simulink model "X-direction-works-UDP"  (R2017a)
settings: Solver=FixedStepDiscrete  StartTime=0.0  StopTime=10.0  FixedStep=0.0002  RelTol=1e-3
libraries: stellaris_lp_lib x7, xpcutilitieslib x2, dspswit3 x1, simulink x1
settings Model: ExtModeTrigDuration=8  Creator=peselnikmg  LastModifiedBy=Rorro
settings DataIOCC: LimitDataPoints=on  SaveFormat=Array  SignalLoggingSaveFormat=ModelDataLogs  ReturnWorkspaceOutputs=on
settings OptimizationCC: UseDivisionForNetSlopeComputation=on  UseFloatMulNetSlope=on  DefaultUnderspecifiedDataType=single  UseSpecifiedMinMax=on  PassReuseOutputArgsAs=Individual arguments  ExpressionDepthLimit=2147483647  ZeroExternalMemoryAtStartup=off  NoFixptDivByZeroProtection=on  EfficientFloat2IntCast=on  LifeSpan=inf  MaxStackSize=64  OptimizeBlockOrder=speed
settings DebuggingCC: ReadBeforeWriteMsg=DisableAll  WriteAfterWriteMsg=DisableAll  WriteAfterReadMsg=DisableAll  MultiTaskDSMMsg=none  IntegerOverflowMsg=error  ParameterTunabilityLossMsg=error  AssertControl=DisableAll  StateNameClashWarn=warning  NonBusSignalsTreatedAsBus=error  SFInvalidInputDataAccessInChartInitDiag=error  SFTransitionOutsideNaturalParentDiag=error  SFUnreachableExecutionPathDiag=error  SFUndirectedBroadcastEventsDiag=error  SFExecutionAtInitializationDiag=none  IntegerSaturationMsg=error
settings HardwareCC: ProdBitPerPointer=32  ProdBitPerSizeT=32  ProdBitPerPtrDiffT=32  ProdLargestAtomicInteger=Long  ProdLargestAtomicFloat=Double  ProdWordSize=32  ProdHWDeviceType=ARM Compatible->ARM Cortex
settings ModelReferenceCC: UpdateModelReferenceTargets=IfOutOfDate  PropagateSignalLabelsOutOfModel=off
settings SFSimCC: SFSimEcho=off  MATLABDynamicMemAlloc=off
settings RTWCC: SystemTargetFile=ert.tlc  HardwareBoard=Tiva TM4C123G Launchpad  TLCOptions=-aInlineSetEventsForThisBaseRateFcn=TLC_FALSE -aSuppressMultiTaskScheduler=TLC_FALSE -aRateBasedStepFcn=1  TemplateMakefile=ert_default_tmf  Description=Embedded Coder  GenerateReport=on  RTWVerbose=off  Toolchain=Texas Instruments Code Composer Studio (Tiva)  IncludeHyperlinkInReport=on  LaunchReport=on  GenerateTraceInfo=on  GenerateTraceReport=on  GenerateTraceReportSl=on  GenerateTraceReportSf=on  GenerateTraceReportEml=on
settings CodeAppCC: ForceParamTrailComments=on  IgnoreCustomStorageClasses=off  OperatorAnnotations=on  SimulinkDataObjDesc=on  SFDataObjDesc=on  MATLABFcnDesc=on  CustomSymbolStrType=$N$R$M  InsertBlockDesc=on  MATLABSourceComments=on  EnableCustomComments=on  ReqsInCode=on
settings ERTTargetCC: UtilityFuncGeneration=Shared location  CombineSignalStateStructs=on  SuppressErrorStatus=on  SupportNonFinite=off  ParenthesesLevel=Maximum  CastingMode=Standards  EnableSignedLeftShifts=off  EnableSignedRightShifts=off
settings ConfigComp: CovMetricSettings=dw  CovHtmlReporting=on  CovSaveCumulativeToWorkspaceVar=on  CovSaveSingleToWorkspaceVar=on  CovExternalEMLEnable=off

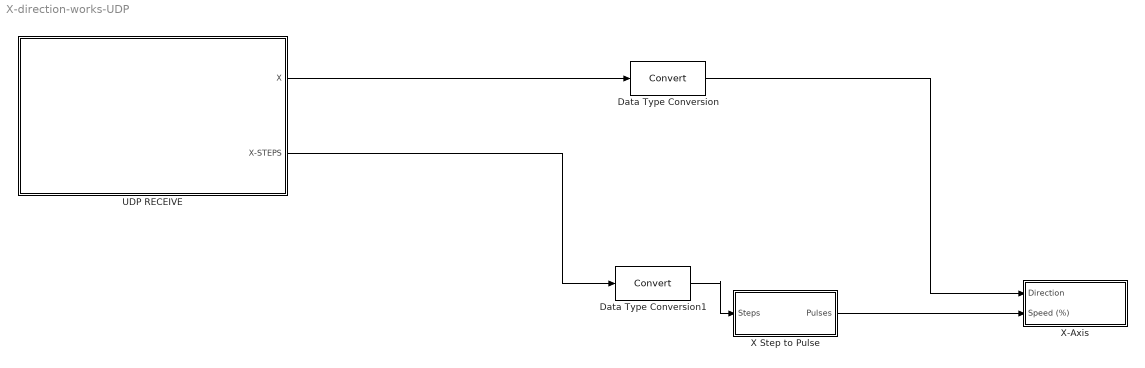
== system X-direction-works-UDP ==
  Data Type Conversion : DataTypeConversion
  Data Type Conversion1 : DataTypeConversion
  UDP RECEIVE : Subsystem
  X Step to Pulse : Subsystem  TreatAsAtomicUnit=on
  X-Axis : Subsystem
  wires:
  X Step to Pulse/1(Pulses) -> X-Axis/2(Speed (%))
  UDP RECEIVE/1(X) -> Data Type Conversion/1
  UDP RECEIVE/2("X-STEPS ") -> Data Type Conversion1/1
  Data Type Conversion/1 -> X-Axis/1(Direction)
  Data Type Conversion1/1 -> X Step to Pulse/1(Steps)

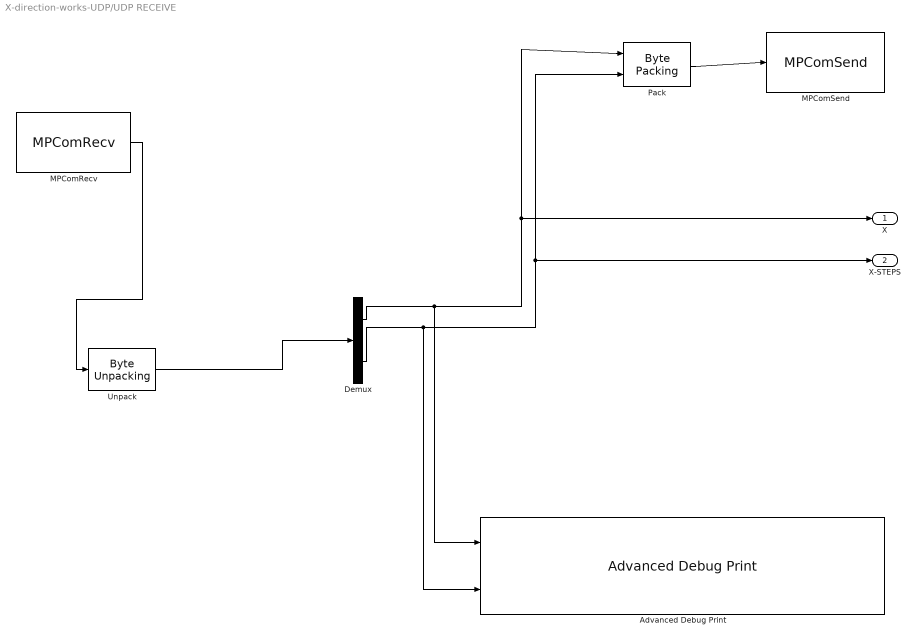
== system X-direction-works-UDP/UDP RECEIVE ==
  Advanced Debug Print : stellaris_lp_lib/Debug/Advanced Debug Print  types={'single','single'}  fmt='X: %hf %hf\r\n'  sample_time=1
      settings: SourceProductName=Run on Stellaris LaunchPad
  Demux : Demux  Outputs=2
  MPComRecv : stellaris_lp_lib/Communication/MPComRecv  vport=2  pack_size=8  sample_time=-1
      settings: SourceProductName=Run on Stellaris LaunchPad
  MPComSend : stellaris_lp_lib/Communication/MPComSend  vport=3  pack_size=8  sample_time=-1
      settings: SourceProductName=Run on Stellaris LaunchPad
  Pack : xpcutilitieslib/Byte Packing   MaskPackedDataType=uint8  MaskUnpackedDataTypes={'single','single'}  MaskAlignment=1
  Unpack : xpcutilitieslib/Byte Unpacking   MaskUnpackedDataTypes={['single']}  MaskUnpackedDataSizes={[1,2]}  MaskAlignment=1
      settings: SourceProductName=Simulink Real-Time  SourceProductBaseCode=XP
  X : Outport
  "X-STEPS " : Outport  Port=2
  wires:
  Demux/1 -> Advanced Debug Print/1, X/1, Pack/1
  Demux/2 -> Advanced Debug Print/2, "X-STEPS "/1, Pack/2
  Pack/1 -> MPComSend/1
  MPComRecv/1 -> Unpack/1
  Unpack/1 -> Demux/1

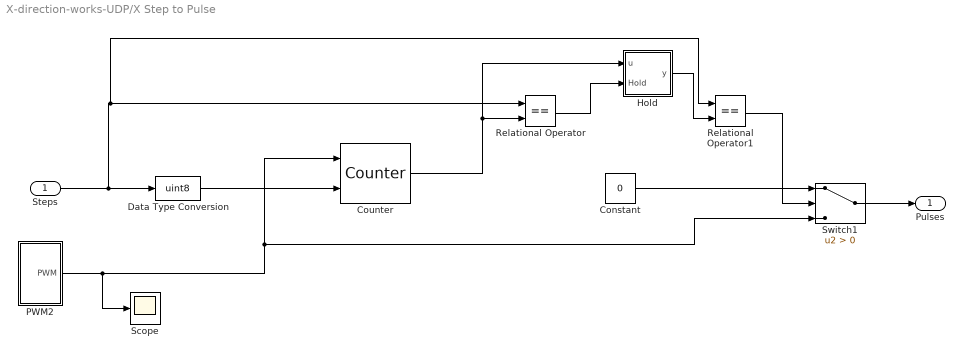
== system X-direction-works-UDP/X Step to Pulse ==
  Steps : Inport
  Constant : Constant  Value=0  OutDataTypeStr=single
  Counter : dspswit3/Counter  Direction=Up  CountEvent=Rising edge  CounterSize=Specify via input port  MaxCount=255  InitialCount=0  Output=Count  HitValue=2  ResetInput=off  SamplesPerFrame=1  Ts=1  CntDtype=single  HitDtype=Logical
  Data Type Conversion : DataTypeConversion  OutDataTypeStr=uint8
  Hold : Subsystem  TreatAsAtomicUnit=on
  PWM2 : Subsystem
  Relational Operator : RelationalOperator  Operator===  OutDataTypeStr=boolean  RndMeth=Simplest
  Relational Operator1 : RelationalOperator  Operator===  OutDataTypeStr=boolean  RndMeth=Simplest
  Scope : Scope
  Switch1 : Switch  Criteria=u2 > Threshold
  Pulses : Outport
  wires:
  Steps/1 -> Relational Operator1/1, Relational Operator/1, Data Type Conversion/1
  Data Type Conversion/1 -> Counter/2
  Relational Operator/1 -> Hold/2(Hold)
  Switch1/1 -> Pulses/1
  Counter/1 -> Hold/1(u), Relational Operator/2
  Constant/1 -> Switch1/1
  PWM2/1(PWM) -> Scope/1, Counter/1, Switch1/3
  Hold/1(y) -> Relational Operator1/2
  Relational Operator1/1 -> Switch1/2

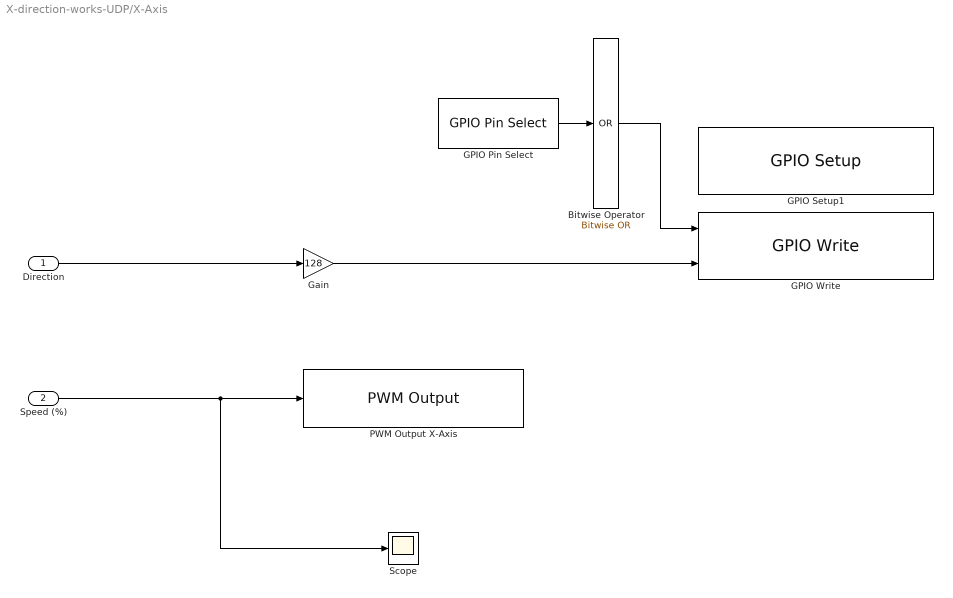
== system X-direction-works-UDP/X-Axis ==
  Direction : Inport  OutDataTypeStr=uint8
  Speed (%) : Inport  Port=2  OutDataTypeStr=single
  Bitwise Operator : simulink/Logic and Bit Operations/Bitwise Operator  logicop=OR  UseBitMask=off  BitMask=bin2dec('11011001')  BitMaskRealWorld=Real World Value
  GPIO Pin Select : stellaris_lp_lib/GPIO/GPIO Pin Select  GPIO_PIN_X=GPIO_PIN_7
      settings: SourceProductName=Run on Stellaris LaunchPad
  GPIO Setup1 : stellaris_lp_lib/GPIO/GPIO Setup  GPIO_PORTX_BASE=GPIO_PORTC_BASE  PinsOutput_0=Unused  PinsOutput_1=Unused  PinsOutput_2=Unused  PinsOutput_3=Unused  PinsOutput_4=Unused  PinsOutput_5=Unused  PinsOutput_6=Unused  PinsOutput_7=Output
      settings: SourceProductName=Run on Stellaris LaunchPad
  GPIO Write : stellaris_lp_lib/GPIO/GPIO Write  GPIO_PORTX_BASE=GPIO_PORTC_BASE  SampleTime=-1
      settings: SourceProductName=Run on Stellaris LaunchPad
  Gain : Gain  Gain=128  ParamDataTypeStr=uint8  OutDataTypeStr=uint8
  PWM Output X-Axis : stellaris_lp_lib/PWM/PWM Output  ch="1    PC4"  invert=off  freq=500  sample_time=-1
      settings: SourceProductName=Run on Stellaris LaunchPad
  Scope : Scope
  wires:
  Direction/1 -> Gain/1
  GPIO Pin Select/1 -> Bitwise Operator/1
  Bitwise Operator/1 -> GPIO Write/1
  Gain/1 -> GPIO Write/2
  Speed (%)/1 -> Scope/1, PWM Output X-Axis/1

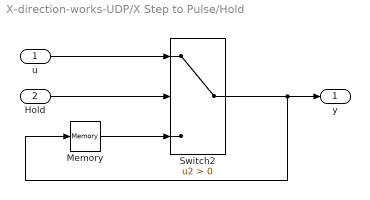
== system X-direction-works-UDP/X Step to Pulse/Hold ==
  u : Inport  OutDataTypeStr=single
  Hold : Inport  Port=2  OutDataTypeStr=boolean
  Memory : Memory
  Switch2 : Switch  Criteria=u2 > Threshold  OutDataTypeStr=single
  y : Outport  OutDataTypeStr=single
  wires:
  u/1 -> Switch2/1
  Switch2/1 -> Memory/1, y/1
  Memory/1 -> Switch2/3
  Hold/1 -> Switch2/2

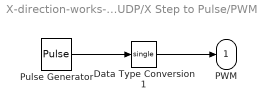
== system X-direction-works-UDP/X Step to Pulse/PWM2 ==
  Data Type Conversion1 : DataTypeConversion  OutDataTypeStr=single
  Pulse Generator : DiscretePulseGenerator  PulseType=Time based  Amplitude=50  Period=.1  PulseWidth=98
  PWM : Outport
  wires:
  Pulse Generator/1 -> Data Type Conversion1/1
  Data Type Conversion1/1 -> PWM/1
